simulink model "dyn_alloc_demo"  (Simulink 8.0)
settings: Solver=ode45  StartTime=0.0  StopTime=10.0  RelTol=1e-3
libraries: qcatlib x1
settings Model: Creator=ola  LastModifiedBy=David  ExtModeAutoUpdateStatusClock=off
settings DataIOCC: SignalLoggingSaveFormat=ModelDataLogs  SignalLoggingName=sigsOut
settings OptimizationCC: BooleanDataType=off
settings DebuggingCC: SaveWithParameterizedLinksMsg=none  SignalResolutionControl=TryResolveAllWithWarning  SolverPrmCheckMsg=none  MultiTaskDSMMsg=warning  MultiTaskCondExecSysMsg=none  StrictBusMsg=None
settings HardwareCC: TargetUnknown=on
settings RTWCC: IncludeERTFirstTime=on
settings GRTTargetCC: CombineOutputUpdateFcns=off  GRTInterface=on

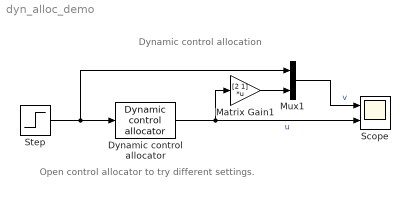
== system dyn_alloc_demo ==
  note: Dynamic control allocation
  note: Open control allocator to try different settings.
  Dynamic control allocator : qcatlib/Dynamic control allocator  B=[2 1]  plim=[-1 1;-1 1]  rlim=[-1 1;-5 5]  T=.1  Wv=1  W1=diag([1 1])  W2=diag([8 0])  S=[.5 0]'
  Matrix Gain1 : Gain  Gain=[2 1]  Multiplication=Matrix(K*u)  SaturateOnIntegerOverflow=on  OutDataTypeStr=Inherit: Same as input  ParamDataTypeStr=Inherit: Same as input
  Mux1 : Mux  Inputs=2
  Scope : Scope  NumInputPorts=2
      settings: TimeRange=10  YMin=0~0  YMax=1.2~1
  Step : Step  SampleTime=0
  wires:
  Matrix Gain1/1 -> Mux1/2
  Dynamic control allocator/1 -> Matrix Gain1/1, Scope/2  "u"
  Mux1/1 -> Scope/1  "v"
  Step/1 -> Mux1/1, Dynamic control allocator/1
